simulink model "KaniewskiHomework2Simulink"  (R2021a)
settings: Solver=VariableStepAuto  StartTime=0.0  StopTime=10  RelTol=1e-3
values from neighbouring files (symbols this model uses):
  F_aileron = dcgain(H_c_inv_aileron)    [hw4script.m]
  F_elevator = dcgain(H_c_inv_elevator)    [hw4script.m]
  F_rudder = dcgain(H_c_inv_rudder)    [hw4script.m]
  F_throttle = dcgain(H_c_inv_throttle)    [hw4script.m]
  Ft = 0.6522    [Homework3Kaniewski.m]
  g = 9.81    [Homework3Kaniewski.m]
  J = [Jxx, 0, 0; 0 Jyy 0; 0 0 Jzz]    [Homework3Kaniewski.m]
  K_A = place(A_A, B_A, [-2,-4,-1])    [hw4script.m]
  K_E = place(A_E, B_E, [-2,-4,-1])    [hw4script.m]
  K_R = place(A_R, B_R, [-2,-4])    [hw4script.m]
  K_T = place(A_T, B_T, [-2,-4])    [hw4script.m]
  m = 0.068    [Homework3Kaniewski.m]
undefined symbols (not defined in the file or in its folder): A_in, E_in, J2, J_inv, M_b_A, R_in, T_in, V_b_0, W_BE_0, Z_inv
libraries: cstblocks x4, vrlib x4
settings Model: Creator=Liza  LastModifiedBy=tomwh
settings DataIOCC: ReturnWorkspaceOutputs=off

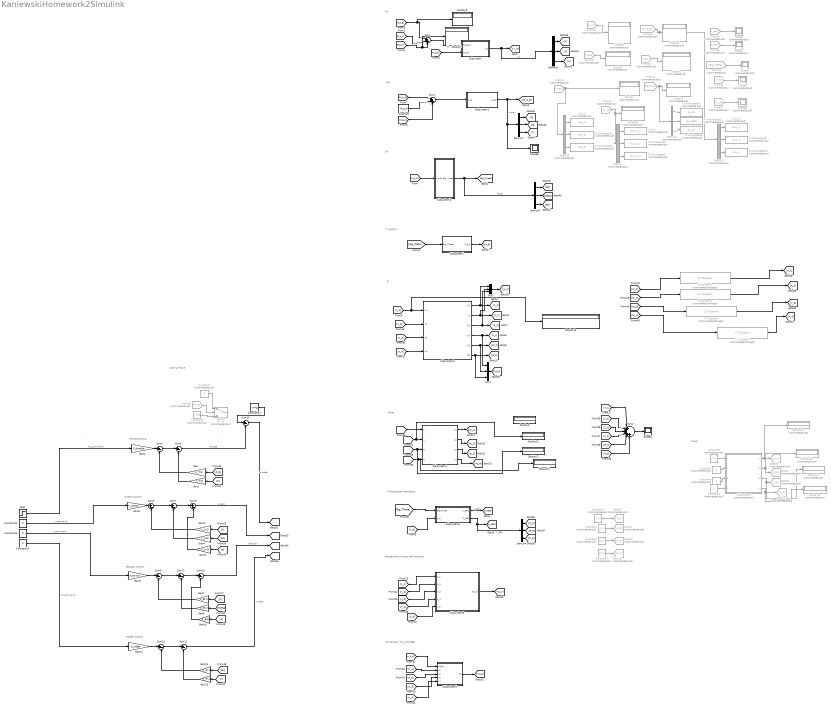
== system KaniewskiHomework2Simulink ==
  note: 5.4
  note: 6.4
  note: 5.5
  note: Translational Kinematics
  note: 7.1 gravity
  note: Mixer
  note: 8
  note: Aerodynamic Forces and Moments
  note: Gyroscopic (M_b_Omega)
  note: Mixer
  note: Throttle Control
  note: Rudder Control
  note: Aileron Control
  note: Elevator Control
  note: Normal Force
  Constant : Constant  Value=M_b_A
  Constant1 : Constant  Commented=on  Value=T_in
  Constant10 : Constant  Commented=on  Value=-m*g
  Constant11 : Constant  Value=-m*g
  Constant12 : Constant  Value=0
  Constant13 : Constant  Value=0
  Constant14 : Constant  Value=0
  Constant2 : Constant  Commented=on  Value=A_in
  Constant3 : Constant  Commented=on  Value=E_in
  Constant4 : Constant  Commented=on  Value=R_in
  Constant{5,7..9} (4 alike) : Constant  Commented=on  Value=0
  Constant6 : Constant  Commented=on  Value=Ft
  Demux{,1..3} (4 alike) : Demux  Commented=on  Outputs=3
  Demux{4..7} (4 alike) : Demux  Outputs=3
  Display{,1..6,14..15,17..18} (11 alike) : Display  Commented=on
  Display{7..13} (7 alike) : Display
  From13 : From  Commented=on  GotoTag=P_NED
  From14 : From  Commented=on  GotoTag=Big_Theta
  From15 : From  Commented=on  GotoTag=V_b
  From16 : From  Commented=on  GotoTag=Big_Theta
  From29 : From  Commented=on  GotoTag=V_NED
  From30 : From  Commented=on  GotoTag=P_NED
  From31 : From  Commented=on  GotoTag=F_b_A
  From32 : From  Commented=on  GotoTag=F_b_g
  From33 : From  Commented=on  GotoTag=F_b_T
  From34 : From  Commented=on  GotoTag=W_b_E
  From40 : From  Commented=on  GotoTag=V_b
  From41 : From  Commented=on  GotoTag=W_b_E
  From60 : From  Commented=on  GotoTag=P_D
  Gain : Gain  Gain=K_T(1)
  Gain1 : Gain  Gain=K_T(2)
  Gain10 : Gain  Gain=K_E(3)
  Gain12 : Gain  Gain=K_R(1)
  Gain13 : Gain  Gain=K_R(2)
  Gain14 : Gain  Gain=F_rudder
  Gain2 : Gain  Gain=F_throttle
  Gain3 : Gain  Gain=K_A(1)
  Gain4 : Gain  Gain=K_A(2)
  Gain5 : Gain  Gain=F_aileron
  Gain6 : Gain  Gain=K_A(3)
  Gain7 : Gain  Gain=K_E(1)
  Gain8 : Gain  Gain=K_E(2)
  Gain9 : Gain  Gain=F_elevator
  Goto20 : Goto  Commented=on  GotoTag=T_in
  Goto21 : Goto  Commented=on  GotoTag=A_in
  Goto22 : Goto  Commented=on  GotoTag=E_in
  Goto23 : Goto  Commented=on  GotoTag=R_in
  Goto24 : Goto  Commented=on  GotoTag=n_1
  Goto25 : Goto  Commented=on  GotoTag=n_3
  Goto26 : Goto  Commented=on  GotoTag=n_4
  Goto27 : Goto  Commented=on  GotoTag=n_2
  LTI System{1..4} (4 alike) : cstblocks/LTI System  Commented=through  sys=tf(15,[1 15],'InputDelay',0.01)  IC=[]
  Mux : Mux  Inputs=3
  Mux1 : Mux  Inputs=3
  Scope{,1,3..5} (5 alike) : Scope  Commented=on
  Scope2 : Scope
  Scope6 : Scope
  Step : Step  Time=5  After=-1  SampleTime=0
  Subsystem : Subsystem
  Subsystem1 : Subsystem
  Subsystem2 : Subsystem
  Subsystem3 : Subsystem
  Subsystem4 : Subsystem
  Subsystem5 : Subsystem
  Subsystem6 : Subsystem
  Subsystem7 : Subsystem
  Subsystem8 : Subsystem
  Subsystem9 : Subsystem  Commented=on
  Sum : Sum  Inputs=|+++
  Sum1 : Sum  Inputs=|+++
  Sum{4..14} (11 alike) : Sum  Inputs=|+-
  Sum2 : Sum  Inputs=|++++++
  Switch : Switch  Commented=on  Criteria=u2 > Threshold
  To Workspace10 : ToWorkspace  Commented=on  VariableName=NLw_r  SaveFormat=Timeseries  SampleTime=0.01
  To Workspace2 : ToWorkspace  Commented=on  VariableName=NLV_b_v  SaveFormat=Timeseries  SampleTime=0.01
  To Workspace3 : ToWorkspace  Commented=on  VariableName=NLV_b_w  SaveFormat=Timeseries  SampleTime=0.01
  To Workspace4 : ToWorkspace  Commented=on  VariableName=NL_phi  SaveFormat=Timeseries  SampleTime=0.01
  To Workspace5 : ToWorkspace  Commented=on  VariableName=NL_theta  SaveFormat=Timeseries  SampleTime=0.01
  To Workspace6 : ToWorkspace  Commented=on  VariableName=NL_psi  SaveFormat=Timeseries  SampleTime=0.01
  To Workspace7 : ToWorkspace  Commented=on  VariableName=NLP_E  SaveFormat=Timeseries  SampleTime=0.01
  To Workspace8 : ToWorkspace  Commented=on  VariableName=NLP_D  SaveFormat=Timeseries  SampleTime=0.01
  To Workspace9 : ToWorkspace  Commented=on  VariableName=NLw_q  SaveFormat=Timeseries  SampleTime=0.01
  V_b_u : ToWorkspace  Commented=on  VariableName=NLV_b_u  SaveFormat=Timeseries  SampleTime=0.01
  V_b_u1 : ToWorkspace  Commented=on  VariableName=NLP_N  SaveFormat=Timeseries  SampleTime=0.01
  V_b_u2 : ToWorkspace  Commented=on  VariableName=NLw_p  SaveFormat=Timeseries  SampleTime=0.01
  wires:
  Sum/1 -> Subsystem/1(Force_b)  "F_b"
  [W_b_E] -> Subsystem/2(W_bE)
  [F_b_A] -> Sum/2
  [F_b_T] -> Display7/1, Sum/3
  [F_b_g] -> Display8/1, Sum/1
  Subsystem/1(v_b) -> Demux5/1, [V_b]  "v_b"
  [M_b_t] -> Sum1/3
  Constant/1 -> Sum1/2
  [n_1] -> Display13/1, Subsystem3/1(n1)
  [n_2] -> Subsystem3/2(n2)
  [n_3] -> Subsystem3/3(n3)
  [n_4] -> Subsystem3/4(n4)
  Subsystem3/1(X_t) -> Mux/1, [X_t]
  Subsystem3/2(Y_t) -> Mux/2, [Y_t]
  Subsystem3/3(Z_t) -> Mux/3, [Z_t]
  Subsystem3/4(L_t) -> Mux1/1, [L_t]
  Subsystem3/5(M_t) -> Mux1/2, [M_t]
  Subsystem3/6(N_t) -> Mux1/3, [N_t]
  Subsystem4/1(n1) -> [nc_1]
  Subsystem4/2(n2) -> [nc_2]
  [W_b_E] -> Subsystem5/1(Wb/e)
  [n_1] -> Subsystem5/2(n1)
  [n_2] -> Subsystem5/3(n2)
  [n_3] -> Subsystem5/4(n3)
  [n_4] -> Subsystem5/5(n4)
  Subsystem5/1(Mb) -> [M_b_O]
  [V_b] -> Subsystem6/5(V_b)
  [n_1] -> Subsystem6/1(n_1)
  [n_4] -> Subsystem6/4(n_4)
  [n_3] -> Subsystem6/3(n_3)
  [n_2] -> Subsystem6/2(n_2)
  Subsystem6/1(F_b_A) -> [F_b_A]
  [Big_Theta] -> Subsystem7/1(Big_Theta)
  Subsystem7/1(F_b_g) -> [F_b_g]
  [Big_Theta] -> Subsystem8/1(Big_Theta)
  [V_b] -> Subsystem8/2(V_b)
  Subsystem8/2(P_NED) -> Demux4/1, [P_NED]  "P_NED"
  Mux/1 -> [F_b_T]
  Mux1/1 -> [M_b_t]
  Subsystem4/3(n3) -> [nc_3]
  Subsystem4/4(n4) -> [nc_4]
  From29/1 -> Scope/1
  From30/1 -> Scope1/1
  From31/1 -> Display1/1
  From32/1 -> Display2/1
  From33/1 -> Display3/1
  Subsystem2/1(Big_Theta) -> Demux6/1, [Big_Theta]  "Theta"
  Subsystem1/1(w_b/E) -> Scope6/1, Demux7/1, [W_b_E]  "w b/e"
  [M_b_O] -> Sum1/1
  Sum1/1 -> Subsystem1/1(M_b)
  [W_b_E] -> Subsystem2/1(w_b/E)
  [X_t] -> Sum2/1
  [Y_t] -> Sum2/2
  [Z_t] -> Sum2/3
  [L_t] -> Sum2/4
  [M_t] -> Sum2/5
  [N_t] -> Sum2/6
  Sum2/1 -> Scope2/1
  Constant1/1 -> Goto20/1
  Constant2/1 -> Goto21/1
  Constant3/1 -> Goto22/1
  Constant4/1 -> Goto23/1
  From14/1 -> Demux1/1, Display5/1
  From15/1 -> Demux/1, Display6/1
  Subsystem8/1(V_NED) -> [V_NED]  "V_NED"
  [Elevator] -> Display11/1, Subsystem4/3(E)
  [Rudder] -> Display12/1, Subsystem4/4(R)
  [Aileron] -> Display10/1, Subsystem4/2(A)
  From16/1 -> Scope3/1
  From40/1 -> Scope4/1
  From41/1 -> Scope5/1
  Demux/1 -> V_b_u/1
  Demux/2 -> To Workspace2/1
  Demux/3 -> To Workspace3/1
  Demux1/1 -> To Workspace4/1
  Demux1/2 -> To Workspace5/1
  Demux1/3 -> To Workspace6/1
  Demux2/2 -> To Workspace7/1
  From13/1 -> Demux2/1, Display/1
  Demux2/3 -> To Workspace8/1
  Demux2/1 -> V_b_u1/1
  Demux3/2 -> To Workspace9/1
  From34/1 -> Demux3/1, Display4/1
  Demux3/3 -> To Workspace10/1
  Demux3/1 -> V_b_u2/1
  Subsystem9/2(n2) -> Display15/1, Goto27/1
  Subsystem9/4(n4) -> Display18/1, Goto26/1
  Subsystem9/1(n1) -> Display14/1, Goto24/1
  Subsystem9/3(n3) -> Display17/1, Goto25/1
  Constant6/1 -> Subsystem9/1(T)
  Constant7/1 -> Subsystem9/2(A)
  Constant8/1 -> Subsystem9/3(E)
  Constant9/1 -> Subsystem9/4(R)
  [nc_1] -> LTI System1/1
  [nc_3] -> LTI System3/1
  [nc_2] -> LTI System2/1
  [nc_4] -> LTI System4/1
  LTI System2/1 -> [n_2]
  LTI System1/1 -> [n_1]
  LTI System3/1 -> [n_3]
  LTI System4/1 -> [n_4]
  Sum10/1 -> Sum11/1
  Gain4/1 -> Sum7/2
  Sum9/1 -> Sum12/1
  Sum8/1 -> [Aileron]  "aileron"
  Gain14/1 -> Sum10/1
  [v] -> Gain3/1
  Gain7/1 -> Sum9/2
  [p] -> Gain6/1
  Constant13/1 -> Gain9/1  "u_command"
  Gain13/1 -> Sum11/2
  [q] -> Gain10/1
  Gain5/1 -> Sum6/1
  Step/1 -> Gain2/1  "P_D_command"
  Gain1/1 -> Sum5/2
  [r] -> Gain13/1
  Gain2/1 -> Sum4/1
  Gain6/1 -> Sum8/2
  [P_D] -> Gain/1
  [u] -> Gain7/1
  Sum4/1 -> Sum5/1
  Sum14/1 -> [Elevator]  "elevator"
  Constant12/1 -> Gain5/1  "v_command"
  Gain/1 -> Sum4/2
  Sum7/1 -> Sum8/1
  Sum12/1 -> Sum14/1
  Sum6/1 -> Sum7/1
  [phi] -> Gain4/1
  [w] -> Gain1/1
  Gain3/1 -> Sum6/2
  Gain10/1 -> Sum14/2
  Sum13/1 -> [Throttle]  "throttle"
  Gain9/1 -> Sum9/1
  Gain8/1 -> Sum12/2
  Sum11/1 -> [Rudder]  "rrudder"
  [theta] -> Gain8/1
  Gain12/1 -> Sum10/2
  [psi] -> Gain12/1
  Sum5/1 -> Sum13/2  "throttle"
  Constant14/1 -> Gain14/1  "psi_command"
  [Throttle] -> Subsystem4/1(T)
  Demux4/1 -> [P_N]
  Demux4/2 -> [P_E]
  Demux4/3 -> [P_D]
  Demux5/1 -> [u]
  Demux5/2 -> [v]
  Demux5/3 -> [w]
  Demux6/1 -> [phi]
  Demux6/2 -> [theta]
  Demux6/3 -> [psi]
  Demux7/1 -> [p]
  Demux7/2 -> [q]
  Demux7/3 -> [r]
  From60/1 -> Switch/2
  Constant5/1 -> Switch/1
  Constant10/1 -> Switch/3
  Constant11/1 -> Sum13/1

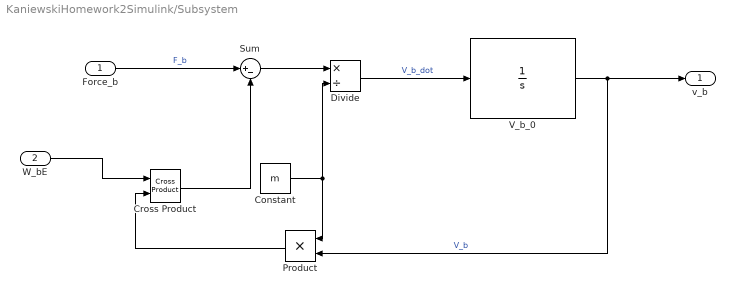
== system KaniewskiHomework2Simulink/Subsystem ==
  Force_b : Inport
  W_bE : Inport  Port=2
  Constant : Constant  Value=m
  Cross Product : vrlib/Utilities/Cross Product
  Divide : Product  Inputs=*/
  Product : Product
  Sum : Sum  Inputs=|+-
  V_b_0 : Integrator  InitialCondition=V_b_0
      settings: AttributesFormatString=%<InitialCondition>
  v_b : Outport
  wires:
  Cross Product/1 -> Sum/2
  V_b_0/1 -> v_b/1, Product/2  "V_b"
  Product/1 -> Cross Product/2
  Force_b/1 -> Sum/1  "F_b"
  Sum/1 -> Divide/1
  W_bE/1 -> Cross Product/1
  Constant/1 -> Product/1, Divide/2
  Divide/1 -> V_b_0/1  "V_b_dot"

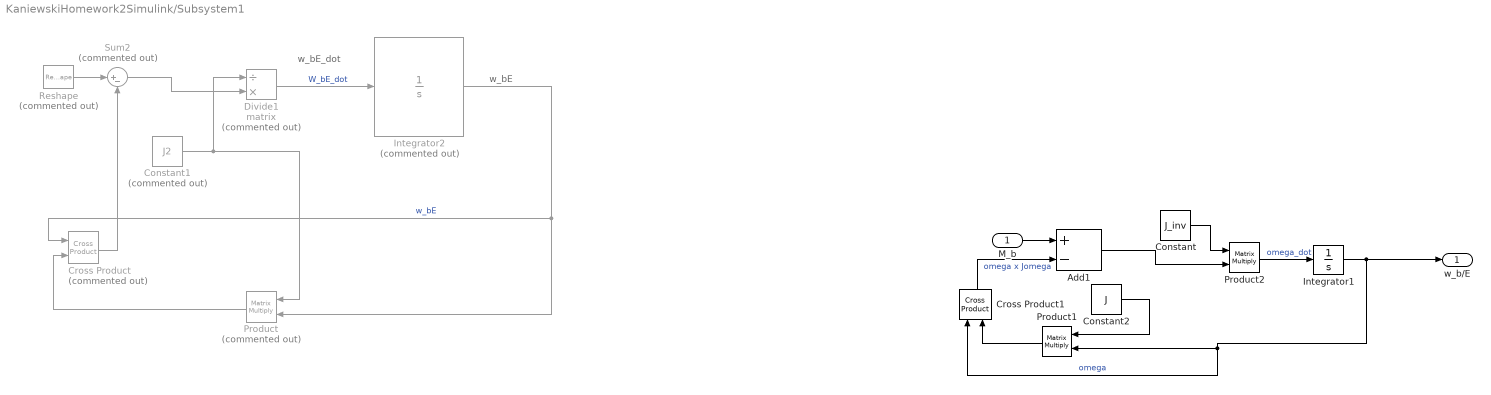
== system KaniewskiHomework2Simulink/Subsystem1 ==
  note: w_bE_dot
  note: w_bE
  M_b : Inport
  Add1 : Sum  Inputs=+-
  Constant : Constant  Value=J_inv
  Constant1 : Constant  Commented=on  Value=J2
  Constant2 : Constant  Value=J
  Cross Product : vrlib/Utilities/Cross Product  Commented=on
  Cross Product1 : vrlib/Utilities/Cross Product
  Divide1 : Product  Commented=on  Inputs=/*  Multiplication=Matrix(*)
  Integrator1 : Integrator  InitialCondition=W_BE_0
      settings: AttributesFormatString=%<InitialCondition>
  Integrator2 : Integrator  Commented=on  InitialCondition=W_BE_0
      settings: AttributesFormatString=%<InitialCondition>
  Product : Product  Commented=on  Multiplication=Matrix(*)
  Product1 : Product  Multiplication=Matrix(*)
  Product2 : Product  Multiplication=Matrix(*)
  Reshape : Reshape  Commented=on  OutputDimensionality=Customize  OutputDimensions=[3,1]
  Sum2 : Sum  Commented=on  Inputs=|+-
  w_b/E : Outport
  wires:
  Constant1/1 -> Divide1/1, Product/1
  Divide1/1 -> Integrator2/1  "W_bE_dot"
  Product/1 -> Cross Product/2
  Sum2/1 -> Divide1/2
  Reshape/1 -> Sum2/1
  Integrator2/1 -> Cross Product/1, Product/2  "w_bE"
  Cross Product/1 -> Sum2/2
  Product1/1 -> Cross Product1/2
  Cross Product1/1 -> Add1/2  "omega x Jomega"
  Product2/1 -> Integrator1/1  "omega_dot"
  Constant2/1 -> Product1/1
  Integrator1/1 -> w_b/E/1, Cross Product1/1, Product1/2  "omega"
  Add1/1 -> Product2/2
  Constant/1 -> Product2/1
  M_b/1 -> Add1/1

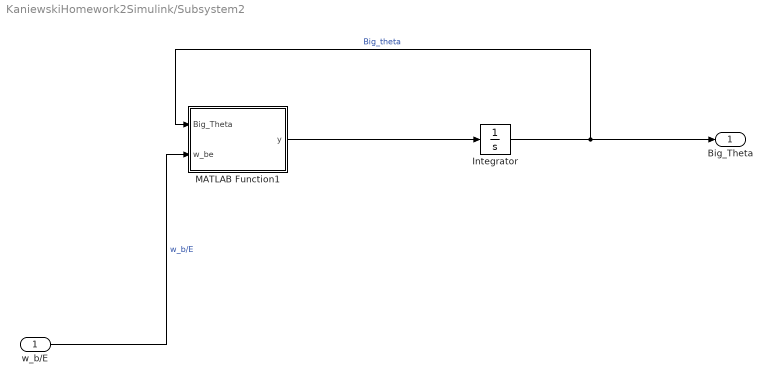
== system KaniewskiHomework2Simulink/Subsystem2 ==
  w_b/E : Inport
  Integrator : Integrator  InitialCondition=[0;0;0];
  MATLAB Function1 : MATLAB Function  TreatAsAtomicUnit=on
  Big_Theta : Outport
  wires:
  w_b/E/1 -> MATLAB Function1/2(w_be)  "w_b/E"
  MATLAB Function1/1(y) -> Integrator/1
  Integrator/1 -> MATLAB Function1/1(Big_Theta), Big_Theta/1  "Big_theta"

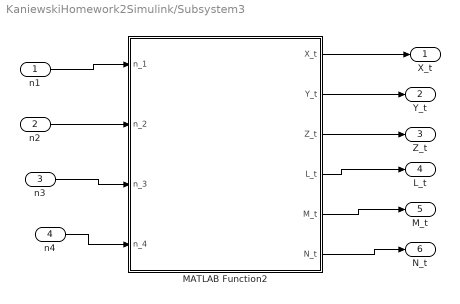
== system KaniewskiHomework2Simulink/Subsystem3 ==
  n1 : Inport
  n2 : Inport  Port=2
  n3 : Inport  Port=3
  n4 : Inport  Port=4
  MATLAB Function2 : MATLAB Function  TreatAsAtomicUnit=on
  X_t : Outport  OutDataTypeStr=double
  Y_t : Outport  Port=2  OutDataTypeStr=double
  Z_t : Outport  Port=3
  L_t : Outport  Port=4
  M_t : Outport  Port=5
  N_t : Outport  Port=6
  wires:
  MATLAB Function2/5(M_t) -> M_t/1
  MATLAB Function2/6(N_t) -> N_t/1
  MATLAB Function2/4(L_t) -> L_t/1
  n1/1 -> MATLAB Function2/1(n_1)
  n2/1 -> MATLAB Function2/2(n_2)
  MATLAB Function2/1(X_t) -> X_t/1
  n3/1 -> MATLAB Function2/3(n_3)
  n4/1 -> MATLAB Function2/4(n_4)
  MATLAB Function2/2(Y_t) -> Y_t/1
  MATLAB Function2/3(Z_t) -> Z_t/1

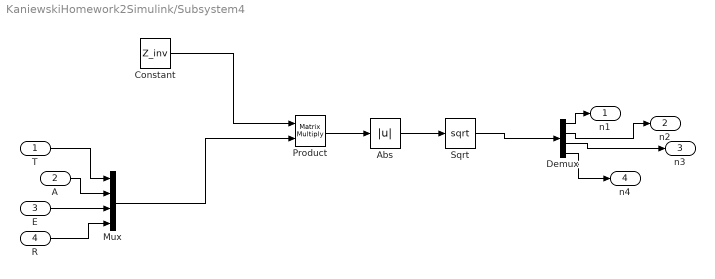
== system KaniewskiHomework2Simulink/Subsystem4 ==
  T : Inport
  A : Inport  Port=2
  E : Inport  Port=3
  R : Inport  Port=4
  Abs : Abs
  Constant : Constant  Value=Z_inv
  Demux : Demux
  Mux : Mux
  Product : Product  Multiplication=Matrix(*)
  Sqrt : Sqrt  SaturateOnIntegerOverflow=on
  n1 : Outport
  n2 : Outport  Port=2
  n3 : Outport  Port=3
  n4 : Outport  Port=4
  wires:
  Abs/1 -> Sqrt/1
  Sqrt/1 -> Demux/1
  Constant/1 -> Product/1
  Mux/1 -> Product/2
  Product/1 -> Abs/1
  T/1 -> Mux/1
  A/1 -> Mux/2
  E/1 -> Mux/3
  R/1 -> Mux/4
  Demux/1 -> n1/1
  Demux/2 -> n2/1
  Demux/3 -> n3/1
  Demux/4 -> n4/1

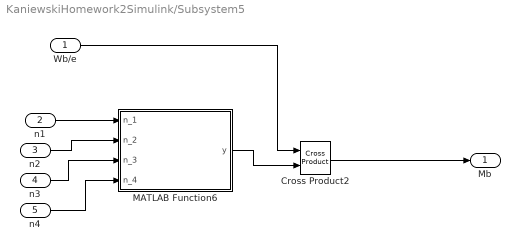
== system KaniewskiHomework2Simulink/Subsystem5 ==
  Wb/e : Inport
  n1 : Inport  Port=2
  n2 : Inport  Port=3
  n3 : Inport  Port=4
  n4 : Inport  Port=5
  Cross Product2 : vrlib/Utilities/Cross Product
  MATLAB Function6 : MATLAB Function  TreatAsAtomicUnit=on
  Mb : Outport
  wires:
  n2/1 -> MATLAB Function6/2(n_2)
  n3/1 -> MATLAB Function6/3(n_3)
  Wb/e/1 -> Cross Product2/1
  n1/1 -> MATLAB Function6/1(n_1)
  n4/1 -> MATLAB Function6/4(n_4)
  MATLAB Function6/1(y) -> Cross Product2/2
  Cross Product2/1 -> Mb/1

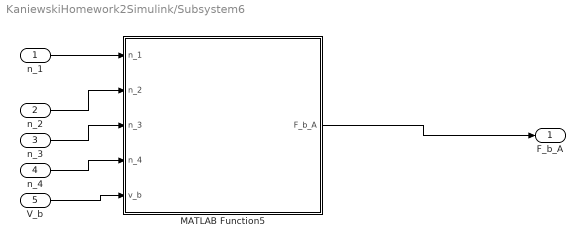
== system KaniewskiHomework2Simulink/Subsystem6 ==
  n_1 : Inport
  n_2 : Inport  Port=2
  n_3 : Inport  Port=3
  n_4 : Inport  Port=4
  V_b : Inport  Port=5
  MATLAB Function5 : MATLAB Function  TreatAsAtomicUnit=on
  F_b_A : Outport
  wires:
  n_3/1 -> MATLAB Function5/3(n_3)
  n_4/1 -> MATLAB Function5/4(n_4)
  n_2/1 -> MATLAB Function5/2(n_2)
  V_b/1 -> MATLAB Function5/5(v_b)
  MATLAB Function5/1(F_b_A) -> F_b_A/1
  n_1/1 -> MATLAB Function5/1(n_1)

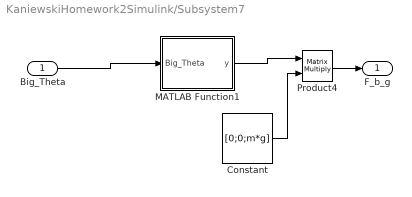
== system KaniewskiHomework2Simulink/Subsystem7 ==
  Big_Theta : Inport
  Constant : Constant  Value=[0;0;m*g]
  MATLAB Function1 : MATLAB Function  TreatAsAtomicUnit=on
  Product4 : Product  Multiplication=Matrix(*)
  F_b_g : Outport
  wires:
  Big_Theta/1 -> MATLAB Function1/1(Big_Theta)
  MATLAB Function1/1(y) -> Product4/1
  Constant/1 -> Product4/2
  Product4/1 -> F_b_g/1

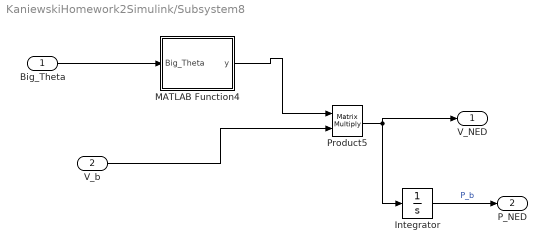
== system KaniewskiHomework2Simulink/Subsystem8 ==
  Big_Theta : Inport
  V_b : Inport  Port=2
  Integrator : Integrator
  MATLAB Function4 : MATLAB Function  TreatAsAtomicUnit=on
  Product5 : Product  Multiplication=Matrix(*)
  V_NED : Outport
  P_NED : Outport  Port=2
  wires:
  Integrator/1 -> P_NED/1  "P_b"
  Product5/1 -> V_NED/1, Integrator/1
  V_b/1 -> Product5/2
  Big_Theta/1 -> MATLAB Function4/1(Big_Theta)
  MATLAB Function4/1(y) -> Product5/1

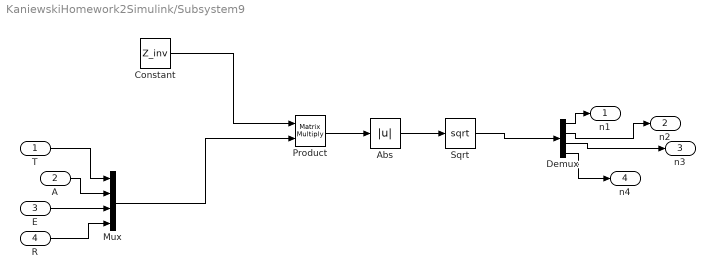
== system KaniewskiHomework2Simulink/Subsystem9 ==
  T : Inport
  A : Inport  Port=2
  E : Inport  Port=3
  R : Inport  Port=4
  Abs : Abs
  Constant : Constant  Value=Z_inv
  Demux : Demux
  Mux : Mux
  Product : Product  Multiplication=Matrix(*)
  Sqrt : Sqrt  SaturateOnIntegerOverflow=on
  n1 : Outport
  n2 : Outport  Port=2
  n3 : Outport  Port=3
  n4 : Outport  Port=4
  wires:
  Abs/1 -> Sqrt/1
  Sqrt/1 -> Demux/1
  Constant/1 -> Product/1
  Mux/1 -> Product/2
  Product/1 -> Abs/1
  T/1 -> Mux/1
  A/1 -> Mux/2
  E/1 -> Mux/3
  R/1 -> Mux/4
  Demux/1 -> n1/1
  Demux/2 -> n2/1
  Demux/3 -> n3/1
  Demux/4 -> n4/1

== matlab function KaniewskiHomework2Simulink/Subsystem7/MATLAB Function1 ==
  data: Big_Theta input; y output
function y = fcn(Big_Theta)
phi = Big_Theta(1);
theta = Big_Theta(2);
psi = Big_Theta(3);
R_phi = [1,0,0;0 cos(phi) sin(phi); 0 -sin(phi) cos(phi)];
R_theta = [cos(theta), 0 -sin(theta); 0 1 0; sin(theta) 0 cos(theta)];
R_psi = [cos(psi) sin(psi) 0; -sin(psi) cos(psi) 0; 0 0 1];
u = R_phi*R_theta*R_psi;
y = u;

== matlab function KaniewskiHomework2Simulink/Subsystem3/MATLAB Function2 ==
  data: X_t output; Y_t output; Z_t output; n_1 input; n_2 input; n_3 input; n_4 input; L_t output; M_t output; N_t output
function [X_t, Y_t, Z_t, L_t, M_t, N_t] = fcn(n_1,n_2,n_3,n_4)
a = 2.0171e-06;
b = 6.7929e-08;
c = 6.7929e-08;
d = 1.0309e-08;

X_t = 0;
Y_t = 0;
Z_t = -a*(n_1^2 + n_2^2 + n_3^2 + n_4^2);
L_t = b*(n_1^2 - n_2^2 - n_3^2 + n_4^2);
M_t = c*(n_1^2 + n_2^2 - n_3^2 - n_4^2);
N_t = d*(-n_1^2 + n_2^2 - n_3^2 + n_4^2);

== matlab function KaniewskiHomework2Simulink/Subsystem8/MATLAB Function4 ==
  data: Big_Theta input; y output
function y = fcn(Big_Theta)
phi = Big_Theta(1);
theta = Big_Theta(2);
psi = Big_Theta(3);
R_b_e =[cos(psi)*cos(theta), cos(psi)*sin(phi)*sin(theta) - cos(phi)*sin(psi), sin(phi)*sin(psi) + cos(phi)*cos(psi)*sin(theta);
cos(theta)*sin(psi), cos(phi)*cos(psi) + sin(phi)*sin(psi)*sin(theta), cos(phi)*sin(psi)*sin(theta) - cos(psi)*sin(phi);
        -sin(theta),                              cos(theta)*sin(phi),                              cos(phi)*cos(theta)];
 



y = R_b_e;

== matlab function KaniewskiHomework2Simulink/Subsystem6/MATLAB Function5 ==
  data: F_b_A output; n_1 input; n_2 input; n_3 input; n_4 input; v_b input
function F_b_A = fcn(n_1,n_2,n_3,n_4,v_b)
Kc = 0.22;
rho = 1.2930;
C_t=0.0822;
D = 0.066;
K = [Kc 0 0;...
    0 Kc 0;...
    0 0 0];
%F_b_A=[0;0;0];
Const = -1*rho*C_t*D^4*(n_1^2 + n_2^2 + n_3^2 + n_4^2);
F_b_A = Const * K* v_b;

== matlab function KaniewskiHomework2Simulink/Subsystem5/MATLAB Function6 ==
  data: n_1 input; y output; n_2 input; n_3 input; n_4 input
function y = fcn(n_1,n_2,n_3,n_4)
J = 0.0270;
u = [0;0;...
    J*2*pi*(n_1-n_2+n_3-n_4)];


y = u;

== matlab function KaniewskiHomework2Simulink/Subsystem2/MATLAB Function1 ==
  data: Big_Theta input; y output; w_be input
function y = fcn(Big_Theta,w_be)
% phi = 0; 
% theta = 0;
% psi = 0;
phi = Big_Theta(1);
theta = Big_Theta(2);
psi = Big_Theta(3);
% phi = 0; 
% theta = 0;
% psi = 0;


A_inv = [1, (sin(phi)*sin(theta))/cos(theta), (cos(phi)*sin(theta))/cos(theta); ...
0,cos(phi), -sin(phi); ...
0,sin(phi)/cos(theta),cos(phi)/cos(theta)];



y = A_inv*w_be;
